simulink model "GNC_sim"  (R2022b)
settings: Solver=VariableStepAuto  StartTime=0.0  StopTime=10.0  RelTol=1e-3
undefined symbols (not defined in the file): A, B, C, D, dT1, dT2, Earth, ELEV_INIT, ELEV_TARGET, K, L, LAT_INIT, LAT_OBS, LAT_TARGET, LON_INIT, LON_OBS, LON_TARGET, Vel, WGS84
libraries: simulink x3, aerolibtransform2 x1, slpidlib x1
settings Model: Creator=matha  LastModifiedBy=matha

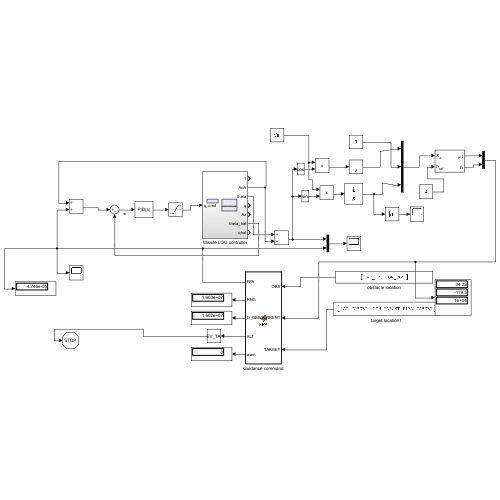
[thumbnail: Simulink's stored preview of the top-level diagram]
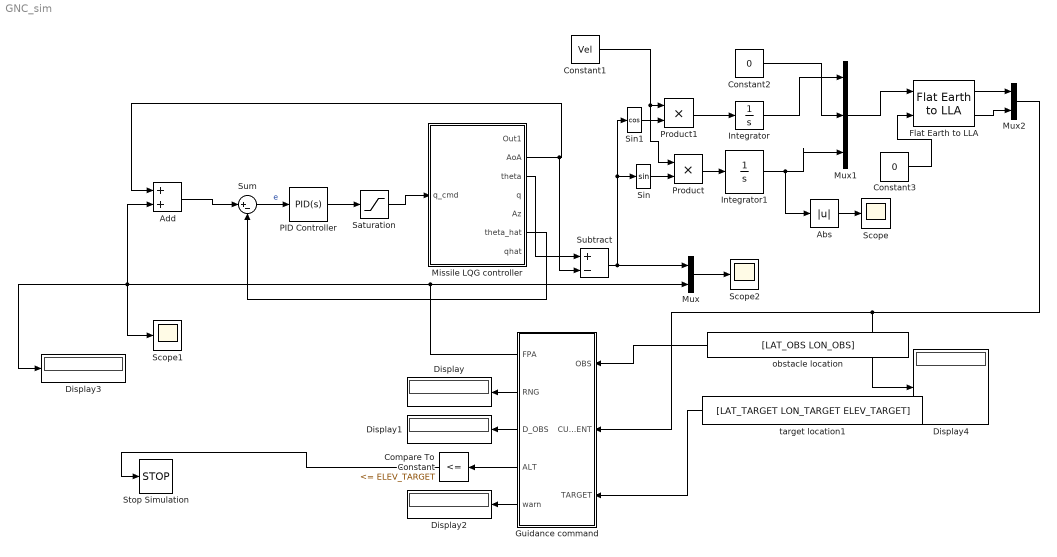
== system GNC_sim ==
  Abs : Abs  SaturateOnIntegerOverflow=off
  Add : Sum
  Compare To Constant : simulink/Logic and Bit Operations/Compare To Constant  relop=<=  const=ELEV_TARGET  OutDataTypeStr=boolean
  Constant1 : Constant  Value=Vel
  Constant2 : Constant  Value=0
  Constant3 : Constant  Value=0
  Display{,1..4} (5 alike) : Display
  Flat Earth to LLA : aerolibtransform2/Flat Earth to LLA  units=Metric (MKS)  ptype=Earth (WGS84)  F=1/298.257223563  R=6378137  refPosPort=off  LL0=[LAT_INIT LON_INIT]  psi=yaw_init
  Guidance command : MATLAB Function  TreatAsAtomicUnit=on
  Integrator : Integrator
  Integrator1 : Integrator  InitialCondition=-ELEV_INIT
  Missile LQG controller : Subsystem
  Mux : Mux  Inputs=2
  Mux1 : Mux  Inputs=3
  Mux2 : Mux  Inputs=2
  PID Controller : slpidlib/PID Controller  Controller=PID  Form=Parallel  TimeDomain=Continuous-time  UseExternalTs=off  SampleTime=-1  IntegratorMethod=Forward Euler  FilterMethod=Forward Euler  ControllerParametersSource=internal  P=-1  I=0  UseKiTs=off  D=1  N=100  UseFilter=on  TunerSelectOption=Transfer Function Based (PID Tuner App)  InitialConditionSource=internal  InitialConditionForIntegrator=0  InitialConditionForFilter=0  DifferentiatorICPrevScaledInput=0  ExternalReset=none  TrackingMode=off  Kt=1  LimitOutput=off  SatLimitsSource=internal  UpperSaturationLimit=inf  LowerSaturationLimit=-inf  LinearizeAsGain=on  AntiWindupMode=none  Kb=1  LimitIntegrator=off  UpperIntegratorSaturationLimit=inf  LowerIntegratorSaturationLimit=-inf  POutMin=[]  POutMax=[]  IOutMin=[]  IOutMax=[]  DOutMin=[]  DOutMax=[]  NOutMin=[]  NOutMax=[]  SumOutMin=[]  SumOutMax=[]  SaturationOutMin=[]  SaturationOutMax=[]  PParamMin=[]  PParamMax=[]  IParamMin=[]  IParamMax=[]  DParamMin=[]  DParamMax=[]  NParamMin=[]  NParamMax=[]  KbParamMin=[]  KbParamMax=[]  KtParamMin=[]  KtParamMax=[]  KbOutMin=[]  KbOutMax=[]  KtOutMin=[]  KtOutMax=[]  IntegratorOutMin=[]  IntegratorOutMax=[]  FilterOutMin=[]  FilterOutMax=[]  SumI1OutMin=[]  SumI1OutMax=[]  SumI2OutMin=[]  SumI2OutMax=[]  SumI3OutMin=[]  SumI3OutMax=[]  SumI4OutMin=[]  SumI4OutMax=[]  SumDOutMin=[]  SumDOutMax=[]  DifferentiatorOutMin=[]  DifferentiatorOutMax=[]  FilterDiffOutCoefMin=[]  FilterDiffOutCoefMax=[]  ReciprocalOutMin=[]  ReciprocalOutMax=[]  SumDenOutMin=[]  SumDenOutMax=[]  SumNumOutMin=[]  SumNumOutMax=[]  DivideOutMin=[]  DivideOutMax=[]  UdiffTsProdOutMin=[]  UdiffTsProdOutMax=[]  NTsProdOutMin=[]  NTsProdOutMax=[]  UintegralTsProdOutMin=[]  UintegralTsProdOutMax=[]  UngainTsProdOutMin=[]  UngainTsProdOutMax=[]  ClampingZeroOutDataTypeStr=Inherit: Inherit via back propagation  ClampingZeroOutMin=[]  ClampingZeroOutMax=[]  FilterDenConstantOutDataTypeStr=Inherit: Inherit via back propagation  FilterDenConstantOutMin=[]  FilterDenConstantOutMax=[]  PCopyOutDataTypeStr=Inherit: Inherit via back propagation  PCopyOutMin=[]  PCopyOutMax=[]  NCopyOutDataTypeStr=Inherit: Inherit via back propagation  NCopyOutMin=[]  NCopyOutMax=[]  IntegratorContinuousStateAttributes=''  IntegratorStateMustResolveToSignalObject=off  IntegratorRTWStateStorageClass=Auto  FilterContinuousStateAttributes=''  FilterStateMustResolveToSignalObject=off  FilterRTWStateStorageClass=Auto  ParallelPVariant=InternalParameters  IdealPVariant=Disabled  IVariant=InternalParameters  DVariant=InternalParameters  IntegratorVariant=Continuous  SatVariant=Disabled  AWVariant=Passthrough  PCopyVariant=Disabled  TRVariant=Disabled  FdbkBlocksVariant=Forward  IdealPFdbkVariant=Disabled  SatFdbkVariant=Disabled  DerivativeFilterVariant=ContFilter  NVariant=InternalParameters  NCopyVariant=Disabled  FilterICVariant=InternalICsFilter  IntegratorICVariant=InternalICs  ExternalResetVariant=Disabled  TRSumVariant=Passthrough  SumFdbkVariant=Disabled  SumVariant=Sum_PID  TsampFilterVariant=InternalTs  TsampNgainVariant=Passthrough  TsampIntegralVariant=Passthrough  ExternalSaturationOutDataTypeStr=Inherit: Same as second input
  Product : Product
  Product1 : Product
  Saturation : Saturate
  Scope : Scope
  Scope1 : Scope
  Scope2 : Scope
  Sin : Trigonometry
  Sin1 : Trigonometry  Operator=cos
  Stop Simulation : Stop
  Subtract : Sum  Inputs=+-
  Sum : Sum  Inputs=|+-
  obstacle location : Constant  Value=[LAT_OBS LON_OBS]
  target location1 : Constant  Value=[LAT_TARGET LON_TARGET ELEV_TARGET]
  wires:
  PID Controller/1 -> Saturation/1
  Saturation/1 -> Missile LQG controller/1(q_cmd)
  Sum/1 -> PID Controller/1  "e"
  Add/1 -> Sum/1
  Missile LQG controller/6(theta_hat) -> Sum/2
  Missile LQG controller/2(AoA) -> Subtract/2, Add/1
  Missile LQG controller/3(theta) -> Subtract/1
  Guidance command/1(FPA) -> Display3/1, Scope1/1, Add/2, Mux/2
  Subtract/1 -> Mux/1, Sin1/1, Sin/1
  Sin/1 -> Product/2
  Sin1/1 -> Product1/2
  Constant1/1 -> Product/1, Product1/1
  Product1/1 -> Integrator/1
  Product/1 -> Integrator1/1
  Integrator/1 -> Mux1/1
  Constant2/1 -> Mux1/2
  Integrator1/1 -> Abs/1, Mux1/3
  Abs/1 -> Scope/1
  Mux1/1 -> Flat Earth to LLA/1
  Constant3/1 -> Flat Earth to LLA/2
  Flat Earth to LLA/1 -> Mux2/1
  Flat Earth to LLA/2 -> Mux2/2
  obstacle location/1 -> Guidance command/1(OBS)
  target location1/1 -> Guidance command/3(TARGET)
  Mux2/1 -> Display4/1, Guidance command/2(CURRENT)
  Guidance command/2(RNG) -> Display/1
  Guidance command/3(D_OBS) -> Display1/1
  Guidance command/5(warn) -> Display2/1
  Guidance command/4(ALT) -> Compare To Constant/1
  Compare To Constant/1 -> Stop Simulation/1
  Mux/1 -> Scope2/1

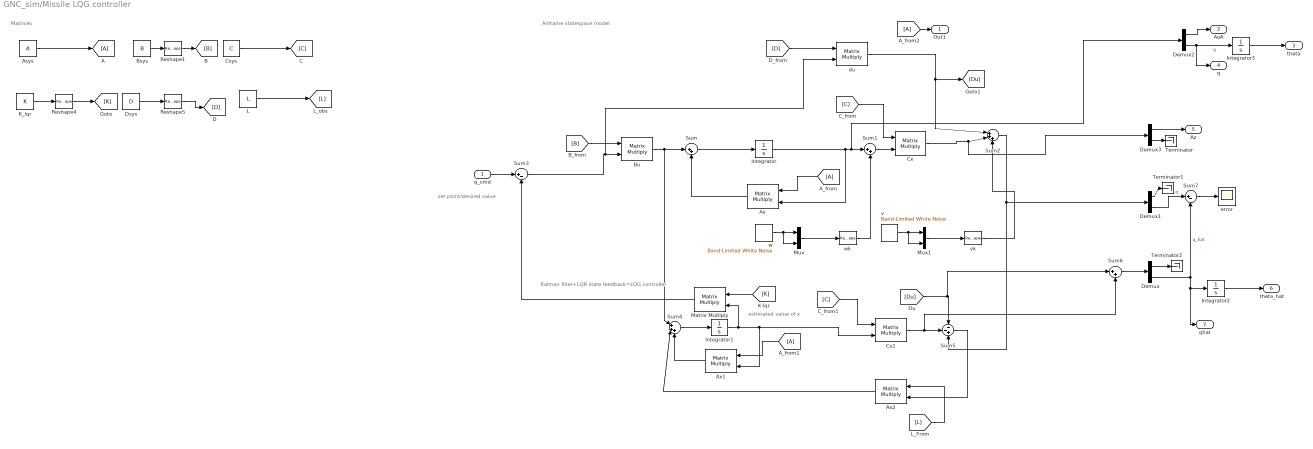
== system GNC_sim/Missile LQG controller ==
  note: set point/desired value
  note: Kalman filter+LQR state feedback=LQG controller
  note: Airframe statespace model
  note: estimated value of x
  note: Matrices
  q_cmd : Inport
  A : Goto
  A_from : From
  A_from1 : From
  A_from2 : From
  Asys : Constant  Value=A
  Ax : Product  Multiplication=Matrix(*)
  Ax1 : Product  Multiplication=Matrix(*)
  Ax2 : Product  Multiplication=Matrix(*)
  Bsys : Constant  Value=B
  Bu : Product  Multiplication=Matrix(*)
  Csys : Constant  Value=C
  Cx : Product  Multiplication=Matrix(*)
  Cx1 : Product  Multiplication=Matrix(*)
  Demux{,1..3} (4 alike) : Demux  Outputs=2
  Dsys : Constant  Value=D
  Integrator{,1..3} (4 alike) : Integrator
  K_lqr : Constant  Value=K
  L : Constant  Value=L
  Matrix Multiply : Product  Multiplication=Matrix(*)
  Mux : Mux  Inputs=2
  Mux1 : Mux  Inputs=2
  Reshape1 : Reshape  OutputDimensionality=Customize  OutputDimensions=[2,1]
  Reshape4 : Reshape  OutputDimensionality=Customize  OutputDimensions=[1,2]
  Reshape5 : Reshape  OutputDimensionality=Customize  OutputDimensions=[2,1]
  Sum : Sum  Inputs=|++
  Sum1 : Sum  Inputs=|++
  Sum2 : Sum  Inputs=|+++
  Sum3 : Sum  Inputs=|+-
  Sum4 : Sum  Inputs=|+++
  Sum5 : Sum  Inputs=--+
  Sum6 : Sum  Inputs=|++
  Sum7 : Sum  Inputs=|+-
  Terminator : Terminator
  Terminator1 : Terminator
  Terminator2 : Terminator
  du : Product  Multiplication=Matrix(*)
  error : Scope
  v : simulink/Sources/Band-Limited White Noise  Cov=[0.00001]  Ts=dT2  seed=[23341]
  vk : Reshape  OutputDimensionality=Customize  OutputDimensions=[2,1]
  w : simulink/Sources/Band-Limited White Noise  Cov=[0.00000001]  Ts=dT1  seed=[23341]
  wk : Reshape  OutputDimensionality=Customize  OutputDimensions=[2,1]
  Out1 : Outport
  AoA : Outport  Port=2
  theta : Outport  Port=3
  q : Outport  Port=4
  Az : Outport  Port=5
  theta_hat : Outport  Port=6
  qhat : Outport  Port=7
  wires:
  Demux3/1 -> Az/1
  Bu/1 -> Sum4/1, Sum/1
  Reshape5/1 -> [D]
  Cx/1 -> Demux3/1, Sum2/2
  du/1 -> Sum2/1, [Du]
  Demux3/2 -> Terminator/1
  Sum6/1 -> Demux/1
  K_lqr/1 -> Reshape4/1
  Bsys/1 -> Reshape1/1
  Demux1/1 -> Terminator1/1
  [B] -> Bu/1
  Sum/1 -> Integrator/1
  [C] -> Cx/1
  vk/1 -> Sum2/3
  Integrator1/1 -> Cx1/2, Ax1/2, Matrix Multiply/2
  Mux/1 -> wk/1
  Integrator/1 -> Ax/2, Demux2/1, Sum1/1
  w/1 -> Mux/2, Mux/1
  wk/1 -> Sum1/2
  Demux/1 -> Terminator2/1
  Sum4/1 -> Integrator1/1
  Demux2/1 -> AoA/1
  A_from1/1 -> Ax1/1
  Asys/1 -> A/1
  [Du] -> Sum6/1, Sum5/1
  A_from2/1 -> Out1/1
  v/1 -> Mux1/2, Mux1/1
  Ax/1 -> Sum/2
  Sum3/1 -> du/2, Bu/2
  Matrix Multiply/1 -> Sum3/2
  [K] -> Matrix Multiply/1
  Cx1/1 -> Sum6/2, Sum5/2
  Demux/2 -> qhat/1, Integrator2/1, Sum7/2  "q_hat"
  Ax2/1 -> Sum4/2
  Demux1/2 -> Sum7/1  "q"
  Dsys/1 -> Reshape5/1
  Demux2/2 -> q/1, Integrator3/1  "q"
  Reshape4/1 -> [K]
  Sum1/1 -> Cx/2
  Sum2/1 -> Demux1/1, Sum5/3
  Mux1/1 -> vk/1
  A_from/1 -> Ax/1
  [D] -> du/1
  Ax1/1 -> Sum4/3
  [C] -> Cx1/1
  Sum7/1 -> error/1
  Integrator3/1 -> theta/1
  Integrator2/1 -> theta_hat/1
  Reshape1/1 -> [B]
  q_cmd/1 -> Sum3/1
  Csys/1 -> [C]
  L/1 -> [L]
  Sum5/1 -> Ax2/2
  [L] -> Ax2/1

== matlab function GNC_sim/Guidance command ==
  data: OBS input; FPA output; CURRENT input; TARGET input; RNG output; D_OBS output; ALT output; warn output
function [FPA,RNG,D_OBS,ALT,warn]= FPA(OBS, CURRENT, TARGET)
%#codegen

R = 6371e3; %earth radius (m)
d2r = pi/180;

%OBSTACLE LOCATION
LAT_OBS = OBS(1);
LON_OBS = OBS(2);

%OBSTACLE THRESHOLD (m)
thres = 2000;

%TARGET location
LAT_TARGET = TARGET(1);
LON_TARGET = TARGET(2);
ELEV_TARGET = TARGET(3); %m - MSL

%CURRENT location
LAT_CUR = CURRENT(2);
LON_CUR = CURRENT(3);
ELEV_CUR = CURRENT(1);

%% distance remaining to target----------------------------------

l1 = LAT_CUR*d2r;
u1 = LON_CUR*d2r;
l2 = LAT_TARGET*d2r;
u2 = LON_TARGET*d2r;
dh = abs(ELEV_TARGET-ELEV_CUR);

dl = l2-l1;
du = u2-u1;

a = sin(dl/2)^2 + cos(l1)*cos(l2)*sin(du/2)^2;
c = 2*atan2(sqrt(a),sqrt(1-a));
d = R*c; %horizontal distance (in m)

%% distance from the obstacle----------------------------------

l3 = LAT_OBS*d2r;
u3 = LON_OBS*d2r;

dl = l3-l1;
du = u3-u1;

a = sin(dl/2)^2 + cos(l1)*cos(l2)*sin(du/2)^2;
c = 2*atan2(sqrt(a),sqrt(1-a));
d_obs = R*c; %horizontal distance (in m)


%% current range (from target) - range > distance
range = sqrt(d^2+dh^2);

%% calculate commanded flight path setpoint - based on d_obs and range

if abs(d_obs)>=thres
    w = 0;
    FPA_CMD = atan(dh/d); %rad
else
    %when <2000m, trigger warning
    w = 1;
    FPA_CMD = 0;
end

%% set output variables

FPA = FPA_CMD;

RNG = range;

D_OBS = d_obs;

warn = w;

ALT = ELEV_CUR;
